simulink model "final_4"  (R2019a)
settings: Solver=FixedStepAuto  StartTime=0.0  StopTime=10  FixedStep=0.0001  RelTol=1e-5
settings Model: Creator=hj823  LastModifiedBy=hj823
settings SolverCC: ShapePreserveControl=EnableAll

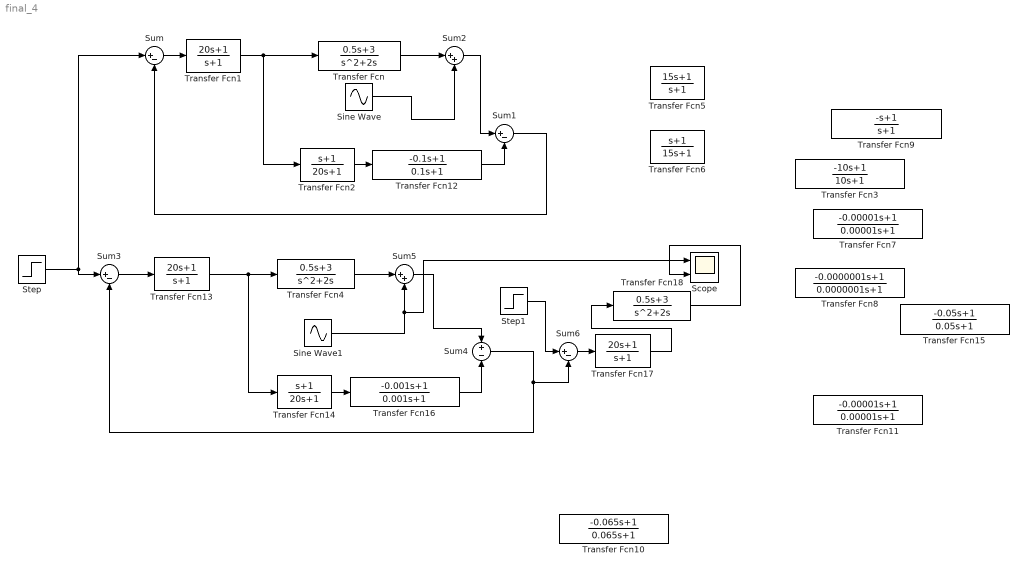
== system final_4 ==
  Scope : Scope  NumInputPorts=2
  Sine Wave : Sin  Amplitude=0.1  Frequency=10  Phase=2.7  SampleTime=0
  Sine Wave1 : Sin  Amplitude=0.1  Frequency=10  Phase=2.7  SampleTime=0
  Step : Step  Before=1  SampleTime=0
  Step1 : Step  Before=1  SampleTime=0
  Sum{,1,3,6} (4 alike) : Sum  Inputs=|+-
  Sum2 : Sum  Inputs=|++
  Sum4 : Sum  Inputs=+-
  Sum5 : Sum  Inputs=|++
  Transfer Fcn : TransferFcn  Numerator=[0.5 3]  Denominator=[1 2 0]
  Transfer Fcn1 : TransferFcn  Numerator=[20 1]  Denominator=[1 1]
  Transfer Fcn10 : TransferFcn  Numerator=[-0.065 1]  Denominator=[0.065 1]
  Transfer Fcn11 : TransferFcn  Numerator=[-0.00001 1]  Denominator=[0.00001 1]
  Transfer Fcn12 : TransferFcn  Numerator=[-0.1 1]  Denominator=[0.1 1]
  Transfer Fcn13 : TransferFcn  Numerator=[20 1]  Denominator=[1 1]
  Transfer Fcn14 : TransferFcn  Numerator=[1 1]  Denominator=[20 1]
  Transfer Fcn15 : TransferFcn  Numerator=[-0.05 1]  Denominator=[0.05 1]
  Transfer Fcn16 : TransferFcn  Numerator=[-0.001 1]  Denominator=[0.001 1]
  Transfer Fcn17 : TransferFcn  Numerator=[20 1]  Denominator=[1 1]
  Transfer Fcn18 : TransferFcn  Numerator=[0.5 3]  Denominator=[1 2 0]
  Transfer Fcn2 : TransferFcn  Numerator=[1 1]  Denominator=[20 1]
  Transfer Fcn3 : TransferFcn  Numerator=[-10 1]  Denominator=[10 1]
  Transfer Fcn4 : TransferFcn  Numerator=[0.5 3]  Denominator=[1 2 0]
  Transfer Fcn5 : TransferFcn  Numerator=[15 1]  Denominator=[1 1]
  Transfer Fcn6 : TransferFcn  Numerator=[1 1]  Denominator=[15 1]
  Transfer Fcn7 : TransferFcn  Numerator=[-0.00001 1]  Denominator=[0.00001 1]
  Transfer Fcn8 : TransferFcn  Numerator=[-0.0000001 1]  Denominator=[0.0000001 1]
  Transfer Fcn9 : TransferFcn  Numerator=[-1 1]  Denominator=[1 1]
  wires:
  Sum2/1 -> Sum1/1
  Sum1/1 -> Sum/2
  Step/1 -> Sum/1, Sum3/1
  Transfer Fcn/1 -> Sum2/1
  Sine Wave/1 -> Sum2/2
  Sum/1 -> Transfer Fcn1/1
  Transfer Fcn1/1 -> Transfer Fcn2/1, Transfer Fcn/1
  Transfer Fcn2/1 -> Transfer Fcn12/1
  Transfer Fcn14/1 -> Transfer Fcn16/1
  Transfer Fcn13/1 -> Transfer Fcn14/1, Transfer Fcn4/1
  Sum5/1 -> Sum4/1
  Transfer Fcn4/1 -> Sum5/1
  Sum3/1 -> Transfer Fcn13/1
  Transfer Fcn12/1 -> Sum1/2
  Sine Wave1/1 -> Scope/1, Sum5/2
  Sum4/1 -> Sum6/2, Sum3/2
  Transfer Fcn16/1 -> Sum4/2
  Step1/1 -> Sum6/1
  Sum6/1 -> Transfer Fcn17/1
  Transfer Fcn17/1 -> Transfer Fcn18/1
  Transfer Fcn18/1 -> Scope/2
